simulink model "qcm_damping"  (R2017b)
settings: Solver=VariableStepAuto  StartTime=0.0  StopTime=sim_time  RelTol=1e-3
values from neighbouring files (symbols this model uses):
  C_max = 5600    [constants18.m]
  C_min = 500    [constants18.m]
  loc = 1    [init.m]
  qcm = struct(qcm)    [constants18.m]
  setV = 0    [init.m]
  your_dut = 18    [init.m]
  Zs0 = [0 0 0 0]    [constants18.m]
  Zu0 = [0 0 0 0]    [constants18.m]
undefined symbols (not defined in the file or in its folder): sigbuilder_block
libraries: simulink x1
settings Model: Creator=rvorster  LastModifiedBy=rvorster

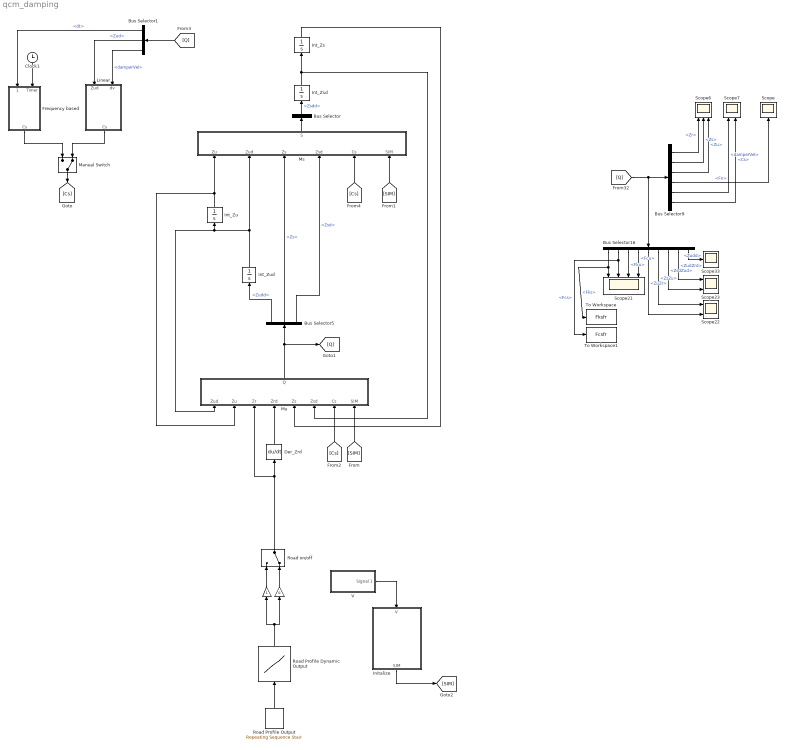
== system qcm_damping ==
  " " : Gain
  " " : Gain  Gain=0
  Bus Selector : BusSelector  OutputSignals=Zsdd
  Bus Selector1 : BusSelector  OutputSignals=dt,Zud,damperVel
  Bus Selector16 : BusSelector  OutputSignals=Fks,Fcs,Fku,Fcu,ZuZr,ZsZu,ZsdZud,ZudZrd,Zudd
  Bus Selector5 : BusSelector  OutputSignals=Zudd,Zs,Zsd
  Bus Selector9 : BusSelector  OutputSignals=Zr,Zs,Zu,Fn,damperVel,Cs
  Clock1 : Clock
  Der_Zrd : Derivative
  Frequency based : Subsystem
  Initalize : MATLAB Function  TreatAsAtomicUnit=on
  Int_Zs : Integrator  InitialCondition=-Zs0(1)
  Int_Zsd : Integrator
  Int_Zu : Integrator  InitialCondition=-Zu0(1)
  Int_Zud : Integrator
  "Linear " : MATLAB Function  TreatAsAtomicUnit=on
  Manual Switch : ManualSwitch  CurrentSetting=0
  Ms : MATLAB Function  TreatAsAtomicUnit=on
  Mu : MATLAB Function  TreatAsAtomicUnit=on
  Road Profile Dynamic Output : Lookup_n-D  NumberOfTableDimensions=1  BreakpointsForDimension1=[-5:5]  Table=tanh([-5:5])  InternalRulePriority=Speed  RndMeth=Simplest  InputSameDT=on
  Road Profile Output : simulink/Sources/Repeating Sequence Stair  OutValues=hx_left  tsamp=time_step  OutMin=[]  OutMax=[]  OutDataTypeStr=double  OutputDataTypeScalingMode=double  OutDataType=fixdt(0,8)  ConRadixGroup=Best Precision: Vector-wise  OutScaling=2^-12
  "Road on/off " : ManualSwitch  CurrentSetting=0
  Scope : Scope
  Scope21 : Scope  NumInputPorts=4
  Scope22 : Scope  NumInputPorts=2
  Scope23 : Scope  NumInputPorts=2
  Scope33 : Scope
  Scope6 : Scope  NumInputPorts=3
  Scope7 : Scope  NumInputPorts=2
  To Workspace : ToWorkspace  VariableName=Fksfr  SaveFormat=Timeseries  SampleTime=-1
  To Workspace1 : ToWorkspace  VariableName=Fcsfr  SaveFormat=Timeseries  SampleTime=-1
  V : Subsystem  Tag=STV Subsys  LoadFcn=sigbuilder_block('load');  StartFcn=sigbuilder_block('start');  StopFcn=sigbuilder_block('stop');  ClipboardFcn=sigbuilder_block('clipboard');  mask(Sigbuilder block){tuvar=[0:10]}
      mask help: Simulink:masks:SigbuilderBlock_MD
      mask init:
      | if ~strcmp(get_param(bdroot(gcbh),'SimulationStatus'),'stopped') tuvar = sigbuilder_block('maskInit'); end
      settings: CopyFcn=sigbuilder_block('copy');  DeleteFcn=sigbuilder_block('delete');  ModelCloseFcn=sigbuilder_block('modelClose');  PreSaveFcn=sigbuilder_block('preSave');  PauseFcn=sigbuilder_block('pause');  ContinueFcn=sigbuilder_block('continue');  NameChangeFcn=sigbuilder_block('namechange');  OpenFcn=sigbuilder_block('open',[433.5 195.75 558 401.25 ]);  CloseFcn=sigbuilder_block('close');
      mask Display: plot(0, 0, 100, 100,[2, 2, 32, 32, 2], [68, 8, 8, 68, 68],[32, 2], [38, 38], [32, 19, 2],[53, 60, 44], [32, 17, 17, 2],[16, 16, 31, 31]);txt = getActiveGroup(gcbh);text(2, 100, txt,'verticalAlignment', 'top');
  wires:
  Int_Zsd/1 -> Mu/6(Zsd), Int_Zs/1
  Int_Zu/1 -> Mu/2(Zu), Ms/1(Zu)
  Bus Selector16/7 -> Scope23/2  "<ZsdZud>"
  Bus Selector16/2 -> To Workspace1/1, Scope21/2  "<Fcs>"
  V/1(Signal 1) -> Initalize/1(V)
  Int_Zs/1 -> Mu/5(Zs)
  [SIM] -> Mu/8(SIM)
  Bus Selector16/3 -> Scope21/3  "<Fku>"
  [Q] -> Bus Selector9/1, Bus Selector16/1
  Initalize/1(SIM) -> [SIM]
  Bus Selector9/5 -> Scope7/1  "<damperVel>"
  Der_Zrd/1 -> Mu/4(Zrd)
  [SIM] -> Ms/6(SIM)
  Bus Selector16/4 -> Scope21/4  "<Fcu>"
  Bus Selector9/2 -> Scope6/2  "<Zs>"
  Bus Selector9/6 -> Scope7/2  "<Cs>"
  Bus Selector16/1 -> To Workspace/1, Scope21/1  "<Fks>"
  Mu/1(Q) -> [Q], Bus Selector5/1
  " "/1 -> "Road on/off "/2
  Bus Selector5/2 -> Ms/3(Zs)  "<Zs>"
  Bus Selector16/8 -> Scope23/1  "<ZudZrd>"
  Ms/1(S) -> Bus Selector/1
  Bus Selector5/3 -> Ms/4(Zsd)  "<Zsd>"
  Bus Selector9/4 -> Scope/1  "<Fn>"
  Bus Selector16/9 -> Scope33/1  "<Zudd>"
  Bus Selector/1 -> Int_Zsd/1  "<Zsdd>"
  Bus Selector9/1 -> Scope6/1  "<Zr>"
  Bus Selector9/3 -> Scope6/3  "<Zu>"
  Bus Selector16/5 -> Scope22/2  "<ZuZr>"
  "Road on/off "/1 -> Mu/3(Zr), Der_Zrd/1
  Int_Zud/1 -> Mu/1(Zud), Int_Zu/1, Ms/2(Zud)
  Bus Selector5/1 -> Int_Zud/1  "<Zudd>"
  Bus Selector16/6 -> Scope22/1  "<ZsZu>"
  " "/1 -> "Road on/off "/1
  Road Profile Dynamic Output/1 -> " "/1, " "/1
  Road Profile Output/1 -> Road Profile Dynamic Output/1
  [Cs] -> Mu/7(Cs)
  [Q] -> Bus Selector1/1
  Bus Selector1/1 -> Frequency based/1("Damper Travel ")  "<dt>"
  Clock1/1 -> Frequency based/2(Timer)
  [Cs] -> Ms/5(Cs)
  Frequency based/1(Cs) -> Manual Switch/1
  Bus Selector1/2 -> "Linear "/1(Zud)  "<Zud>"
  "Linear "/1(Cs) -> Manual Switch/2
  Manual Switch/1 -> [Cs]
  Bus Selector1/3 -> "Linear "/2(dv)  "<damperVel>"

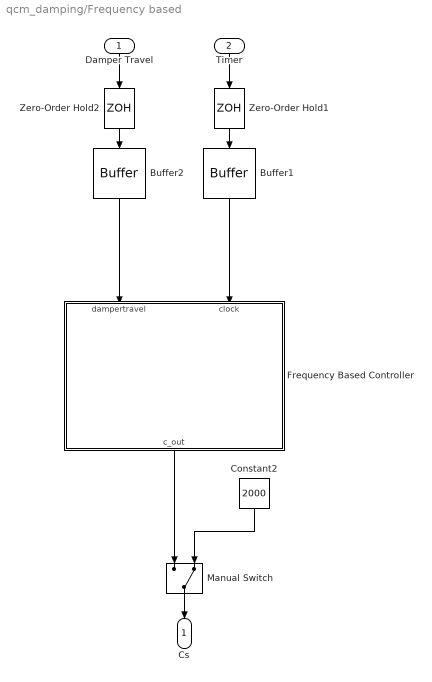
== system qcm_damping/Frequency based ==
  "Damper Travel " : Inport
  Timer : Inport  Port=2
  Buffer1 : Buffer  N=50  OutputFrames=off
  Buffer2 : Buffer  N=50  OutputFrames=off
  Constant2 : Constant  Value=2000
  Frequency Based Controller : MATLAB Function  TreatAsAtomicUnit=on
  Manual Switch : ManualSwitch  CurrentSetting=0
  Zero-Order Hold1 : ZeroOrderHold  SampleTime=1000
  Zero-Order Hold2 : ZeroOrderHold
  Cs : Outport
  wires:
  Frequency Based Controller/1(c_out) -> Manual Switch/1
  Manual Switch/1 -> Cs/1
  Constant2/1 -> Manual Switch/2
  Zero-Order Hold2/1 -> Buffer2/1
  Buffer2/1 -> Frequency Based Controller/1(dampertravel)
  "Damper Travel "/1 -> Zero-Order Hold2/1
  Buffer1/1 -> Frequency Based Controller/2(clock)
  Zero-Order Hold1/1 -> Buffer1/1
  Timer/1 -> Zero-Order Hold1/1

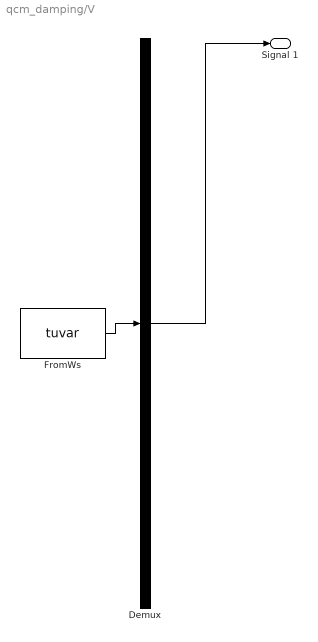
== system qcm_damping/V ==
  Demux : Demux  Tag=STV Demux  Outputs=1
  FromWs : FromWorkspace  Tag=STV FromWs  VariableName=tuvar  SampleTime=0
      SigBuilderData=|
      | common.afterFinalStr = 'Extrapolate'
      | common.sampleTime = 0
      | dataSet.timeRange = [0 10]
      | dataSet.name = 'Group 1'
      | sbobj.Groups.Name = 'Group 1'
      | sbobj.Groups.Signals.Name = 'Signal 1'
      | sbobj.Groups.Signals.XData = [0 4 6 10]
      | sbobj.Groups.Signals.YData = [0 35 0 0]
  Signal 1 : Outport  Tag=STV Outport
  wires:
  Demux/1 -> Signal 1/1
  FromWs/1 -> Demux/1

== matlab function qcm_damping/Ms ==
  data: Zu input; Zud input; Zs input; Zsd input; Cs input; SIM input Bus: SIM; S output Bus: C; qcm parameter; loc parameter
function S = fcm(Zu, Zud, Zs, Zsd, Cs, SIM, qcm, loc)

    S = sprung_mass_damper_in(Zu, Zud, Zs, Zsd, Cs, SIM, loc, qcm);
    
end

== matlab function qcm_damping/Mu ==
  data: Zud input; Zu input; Zr input; Zrd input; Q output Bus: U; Zs input; Zsd input; Cs input; qcm parameter; loc parameter; SIM input Bus: SIM; Zs0 parameter
function Q = fcn(Zud, Zu, Zr, Zrd, Zs, Zsd, Cs, qcm, loc, SIM, Zs0)

    Q = unsprung_mass_damper_in(Zud, Zu, Zrd, Zr, Zsd, Zs, Cs, loc, SIM, Zs0, qcm);

end

== matlab function qcm_damping/Frequency based/Frequency Based Controller ==
  data: dampertravel input; c_out output; clock input
function c_out   = fcn(dampertravel, clock)
x = dampertravel;
t = clock;

dt = t(end) - t(end - 1);% gets time step there FIXED STEPS ONLY IN SIMULINK
fs = 1/dt; % sampling frequency
startindex = t(1);

totindexnum = length(t);

bins = t*fs - startindex + 1;
fHz = bins*fs/totindexnum;

X = fft(x);
X_mag = abs(X);

% 	startfirstrangeindex = find(fHz == 1, 1, 'last');
% 	endfirstrangeindex = find(fHz == 5, 1, 'last');
% 
% 	startsecondrangeindex = find(fHz ==5, 1, 'last');
% 	endsecondrangeindex = find(fHz == 20, 1, 'last');
startfirstrangeindex = (1*totindexnum)/fs;
endfirstrangeindex = (5*totindexnum)/fs;
% 	endfirstrangeindex = 2;

% 	startsecondrangeindex = 2;
% 	endsecondrangeindex = 8;
startsecondrangeindex = (5*totindexnum)/fs;
endsecondrangeindex = (20*totindexnum)/fs;

if startfirstrangeindex + endfirstrangeindex ~= 0

	area1 = trapz(X_mag(startfirstrangeindex:endfirstrangeindex));
	area2 = trapz(X_mag(startsecondrangeindex:endsecondrangeindex));

	if area1/area2 >= 0.1
		c_out = 5000;
	elseif area1/area2 < 0.1
		c_out = 200;
	else	
		c_out = 8000;
	end
else
	c_out = 2000;
end

== matlab function qcm_damping/Linear  ==
  data: Zud input; dv input; Cs output; C_max parameter; C_min parameter
function Cs = fcn(Zud, dv, C_max, C_min)

if Zud*dv >= 0
    Cs = C_max;	
	
elseif Zud*dv < 0
    Cs = C_min;
else
    Cs = 2000;
end

== matlab function qcm_damping/Initalize ==
  settings: updateMethod=DISCRETE
  data: V input; qcm parameter; SIM output Bus: SIM; setV parameter; loc parameter; your_dut parameter
function SIM = fcn(V, qcm, setV, loc, your_dut)

    if (setV == 0)
        SIM.V = qcm.V;
        SIM.L = 0.5*qcm.V^2*qcm.ClA*qcm.rho0;
        SIM.sim_time = 0;
        SIM.sim_step = 0;
        SIM.time_step = 0.01 / qcm.V;
        SIM.your_dut = your_dut;
        SIM.loc = loc;
    else
        SIM.V = V;
        SIM.L = 0.5*V^2*qcm.ClA*qcm.rho0;
        SIM.sim_time = 0;
        SIM.sim_step = 0;
        SIM.time_step = 0.01 / V;
        SIM.your_dut = your_dut;
        SIM.loc = loc;
    end

end
